simulink model "task1"  (R2018a)
settings: Solver=FixedStepAuto  StartTime=0.0  StopTime=20  FixedStep=1e-3  MaxStep=1e-3  RelTol=1e-3
libraries: powerlib_meascontrol x1
settings Model: Creator=User  LastModifiedBy=User

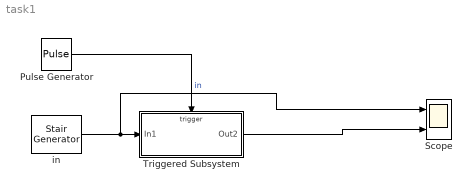
== system task1 ==
  Pulse Generator : DiscretePulseGenerator  PulseType=Time based  Period=1  PulseWidth=25  PhaseDelay=0.01
  Scope : Scope  NumInputPorts=2
  Triggered Subsystem : Subsystem  TreatAsAtomicUnit=on
  in : powerlib_meascontrol/Pulse & Signal Generators/Stair Generator  t=time  e=in  Ts=0
      settings: SourceProductName=Simscape Power Systems
  wires:
  in/1 -> Scope/1, Triggered Subsystem/1(In1)  "in"
  Pulse Generator/1 -> Triggered Subsystem/Trigger
  Triggered Subsystem/1(Out2) -> Scope/2

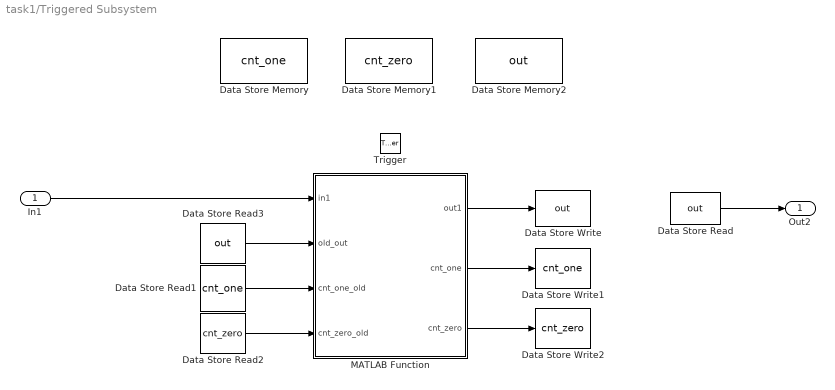
== system task1/Triggered Subsystem ==
  In1 : Inport
  Trigger : TriggerPort  VariantControl=Variant  InitialTriggerSignalState=positive
  Data Store Memory : DataStoreMemory  DataStoreName=cnt_one  ReadBeforeWriteMsg=warning  WriteAfterWriteMsg=warning  WriteAfterReadMsg=warning  ShowAdditionalParam=off
  Data Store Memory1 : DataStoreMemory  DataStoreName=cnt_zero  ReadBeforeWriteMsg=warning  WriteAfterWriteMsg=warning  WriteAfterReadMsg=warning  ShowAdditionalParam=off
  Data Store Memory2 : DataStoreMemory  DataStoreName=out  ReadBeforeWriteMsg=warning  WriteAfterWriteMsg=warning  WriteAfterReadMsg=warning  ShowAdditionalParam=off
  Data Store Read : DataStoreRead  DataStoreName=out
  Data Store Read1 : DataStoreRead  DataStoreName=cnt_one
  Data Store Read2 : DataStoreRead  DataStoreName=cnt_zero
  Data Store Read3 : DataStoreRead  DataStoreName=out
  Data Store Write : DataStoreWrite  DataStoreName=out
  Data Store Write1 : DataStoreWrite  DataStoreName=cnt_one
  Data Store Write2 : DataStoreWrite  DataStoreName=cnt_zero
  MATLAB Function : MATLAB Function  TreatAsAtomicUnit=on
  Out2 : Outport
  wires:
  In1/1 -> MATLAB Function/1(in1)
  MATLAB Function/1(out1) -> Data Store Write/1
  Data Store Read1/1 -> MATLAB Function/3(cnt_one_old)
  Data Store Read2/1 -> MATLAB Function/4(cnt_zero_old)
  MATLAB Function/2(cnt_one) -> Data Store Write1/1
  Data Store Read3/1 -> MATLAB Function/2(old_out)
  Data Store Read/1 -> Out2/1
  MATLAB Function/3(cnt_zero) -> Data Store Write2/1

== matlab function task1/Triggered Subsystem/MATLAB Function ==
  data: in1 input; old_out input; out1 output; cnt_one_old input; cnt_zero_old input; cnt_one output; cnt_zero output
function [out1, cnt_one, cnt_zero] = fcn(in1, old_out, cnt_one_old, cnt_zero_old)
if in1 == 0 && cnt_one_old ==0 %Ждем 1, для начала серии
  cnt_one = 0;
  cnt_zero = 0;
  out1 = old_out;    
elseif in1 == 1 % Если на входе 1, счетчик единиц инкрементируем, остальнео без изменений
  cnt_one = cnt_one_old + 1;
  cnt_zero = 0;
  out1 = old_out;
elseif cnt_zero_old == 0 %Если на входе 0, но еще не было двух подряд, то инкрементируем счетчик нулей
  cnt_zero = cnt_zero_old +1;
  out1 = old_out;
  cnt_one = cnt_one_old + 0;
elseif mod(cnt_one_old,2) == 0 %Если два нуля подряд, то, если единиц нечетное кол-во, выход 0, иначе 1. Сбрасываем счетчики
  out1 = 1;
  cnt_one = 0;
  cnt_zero = 0;
else
  out1 = 0;
  cnt_one = 0;
  cnt_zero = 0; 
end
